simulink model "single_phase_bridge_hc"  (Simulink 6.1)
settings: Solver=ode23tb  StartTime=0.0  StopTime=0.3  MaxStep=1e-4  RelTol=1e-3  AbsTol=.01
libraries: powerlib x10
settings Model: LastModifiedBy=ThinkPad
settings DebuggingCC: SolverPrmCheckMsg=warning

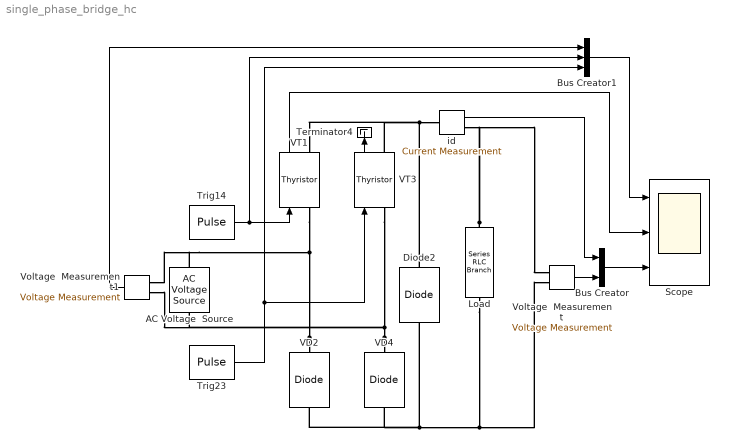
== system single_phase_bridge_hc ==
  AC Voltage  Source : powerlib/Electrical Sources/AC Voltage Source  Orientation=up  Amplitude=100  Phase=0  Frequency=50  SampleTime=0  Measurements=None
  Bus Creator : BusCreator  DialogController=Simulink.DDGSource_Bus  Inputs=2
  Bus Creator1 : BusCreator  DialogController=Simulink.DDGSource_Bus  Inputs=3
  Diode2 : powerlib/Power Electronics/Diode  Orientation=up  Ron=0.001  Lon=0  Vf=0.8  IC=0  Rs=500  Cs=250e-9  Measurements=off
  Load : powerlib/Elements/Series RLC Branch  Orientation=down  PhysicalDomain=powersysdomain  SubClassName=unknown  LeftPortType=p1  RightPortType=p1  LConnTagsString=__new0  RConnTagsString=__new0  Resistance=1  Inductance=0.1  Capacitance=inf  Measurements=None
  Scope : Scope  NumInputPorts=3
      settings: TimeRange=0.1  YMin=-100~-100~0  YMax=100~100~100  Decimation=5  SampleInput=on  SampleTime=1e-4
  Terminator4 : Terminator
      settings: Orientation=up
  Trig14 : DiscretePulseGenerator  PulseType=Time based  Amplitude=10  Period=0.02  PulseWidth=5  PhaseDelay=0.0025
  Trig23 : DiscretePulseGenerator  PulseType=Time based  Amplitude=10  Period=0.02  PulseWidth=5  PhaseDelay=0.0125
  VD2 : powerlib/Power Electronics/Diode  Orientation=up  Ron=0.001  Lon=0  Vf=0.8  IC=0  Rs=500  Cs=250e-9  Measurements=off
  VD4 : powerlib/Power Electronics/Diode  Orientation=up  Ron=0.001  Lon=0  Vf=0.8  IC=0  Rs=500  Cs=250e-9  Measurements=off
  VT1 : powerlib/Power Electronics/Thyristor  Orientation=up  Ron=0.01  Lon=0  Vf=0.8  IC=0  Rs=1000  Cs=100e-9  Measurements=on
  VT3 : powerlib/Power Electronics/Thyristor  Orientation=up  Ron=0.01  Lon=0  Vf=0.8  IC=0  Rs=1000  Cs=100e-9  Measurements=on
  Voltage  Measurement : powerlib/Measurements/Voltage Measurement  PhasorSimulation=off  OutputType=Complex  PSBequivalent=0
  Voltage  Measurement1 : powerlib/Measurements/Voltage Measurement  Orientation=left  PhasorSimulation=off  OutputType=Complex  PSBequivalent=0
  id : powerlib/Measurements/Current Measurement  PhasorSimulation=off  OutputType=Complex  PSBequivalent=0
  wires:
  Trig14/1 -> Bus Creator1/2, VT1/1
  VT1/1 -> Scope/2
  Voltage  Measurement/1 -> Bus Creator/2
  Bus Creator/1 -> Scope/3
  id/1 -> Bus Creator/1
  Trig23/1 -> VT3/1, Bus Creator1/3
  Bus Creator1/1 -> Scope/1
  Voltage  Measurement1/1 -> Bus Creator1/1
  VT3/1 -> Terminator4/1
  connections:
  id/RConn1 -- Load/LConn1 -- Voltage  Measurement/LConn1
  VT3/RConn1 -- VT1/RConn1 -- id/LConn1 -- Diode2/RConn1
  VD2/LConn1 -- VD4/LConn1 -- Voltage  Measurement/LConn2 -- Load/RConn1 -- Diode2/LConn1
  VD4/RConn1 -- Voltage  Measurement1/LConn2 -- AC Voltage  Source/LConn1 -- VT3/LConn1
  VD2/RConn1 -- Voltage  Measurement1/LConn1 -- AC Voltage  Source/RConn1 -- VT1/LConn1
